simulink model "Motor_C_mex"  (R2024a)
settings: Solver=FixedStepAuto  StartTime=0.0  StopTime=20  FixedStep=MotorSampleTime  RelTol=1e-3
model workspace (MAT data in the model file):
  MotorSampleTime = 0.001
undefined symbols (not defined in the file): DiscIntNeverNeededParam
libraries: sldrtlib x1
settings Model: SimulationMode=accelerator  Creator=17739  LastModifiedBy=17739

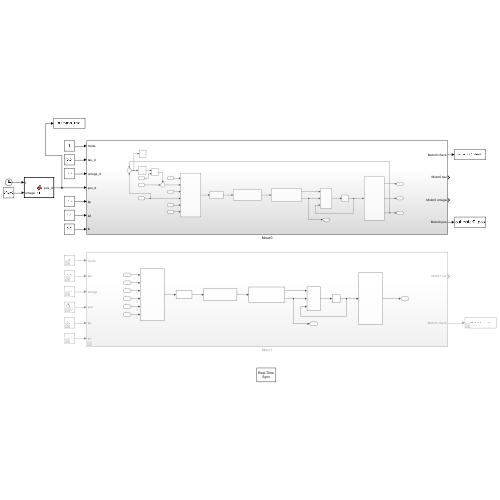
[thumbnail: Simulink's stored preview of the top-level diagram]
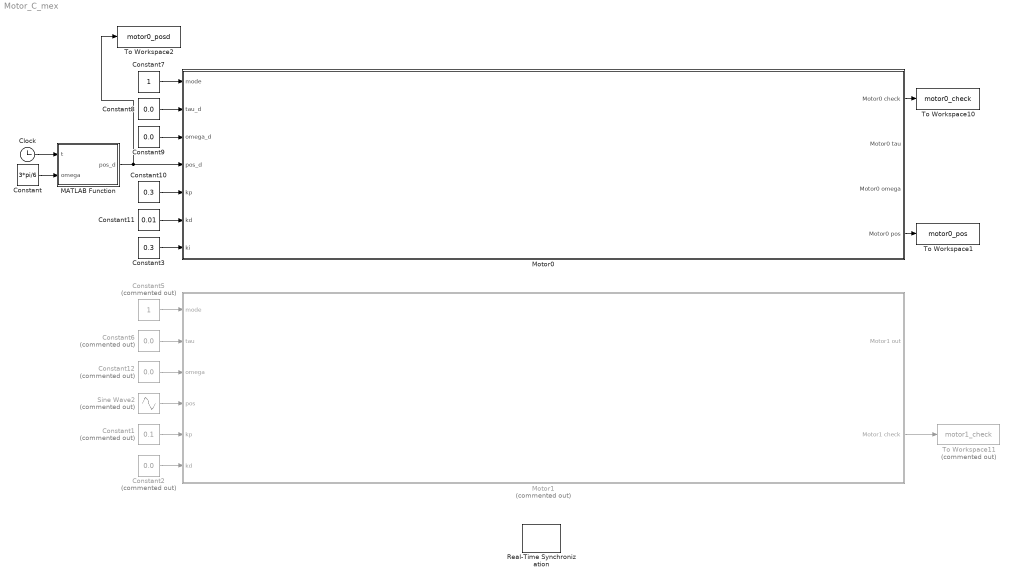
== system Motor_C_mex ==
  Clock : Clock
  Constant : Constant  Value=3*pi/6
  Constant1 : Constant  Commented=on  Value=0.1
  Constant10 : Constant  Value=0.3
  Constant11 : Constant  Value=0.01
  Constant12 : Constant  Commented=on  Value=0.0
  Constant2 : Constant  Commented=on  Value=0.0
  Constant3 : Constant  Value=0.3
  Constant5 : Constant  Commented=on
  Constant6 : Constant  Commented=on  Value=0.0
  Constant7 : Constant
  Constant8 : Constant  Value=0.0
  Constant9 : Constant  Value=0.0
  MATLAB Function : MATLAB Function  TreatAsAtomicUnit=on
  Motor0 : Subsystem
  Motor1 : Subsystem  Commented=on
  Real-Time Synchronization : sldrtlib/Real-Time Synchronization  SampleTime=MotorSampleTime  MaxMissedTicks=inf  ShowMissedTicks=off  YieldWhenWaiting=off
  Sine Wave2 : Sin  Commented=on  Amplitude=pi*6.33  Frequency=pi/5  SampleTime=MotorSampleTime
  To Workspace1 : ToWorkspace  VariableName=motor0_pos  SampleTime=-1
  To Workspace10 : ToWorkspace  VariableName=motor0_check  SampleTime=-1
  To Workspace11 : ToWorkspace  Commented=on  VariableName=motor1_check  SampleTime=-1
  To Workspace2 : ToWorkspace  VariableName=motor0_posd  SampleTime=-1
  wires:
  Constant7/1 -> Motor0/1(mode)
  Constant10/1 -> Motor0/5(kp)
  Motor1/2(Motor1 check) -> To Workspace11/1
  Constant8/1 -> Motor0/2(tau_d)
  Constant5/1 -> Motor1/1(mode)
  Constant2/1 -> Motor1/6(kd)
  Constant6/1 -> Motor1/2(tau)
  Constant11/1 -> Motor0/6(kd)
  Motor0/1(Motor0 check) -> To Workspace10/1
  Constant9/1 -> Motor0/3(omega_d)
  Constant1/1 -> Motor1/5(kp)
  Sine Wave2/1 -> Motor1/4(pos)
  Constant12/1 -> Motor1/3(omega)
  Constant3/1 -> Motor0/7(ki)
  Motor0/4(Motor0 pos) -> To Workspace1/1
  MATLAB Function/1(pos_d) -> To Workspace2/1, Motor0/4(pos_d)
  Clock/1 -> MATLAB Function/1(t)
  Constant/1 -> MATLAB Function/2(omega)

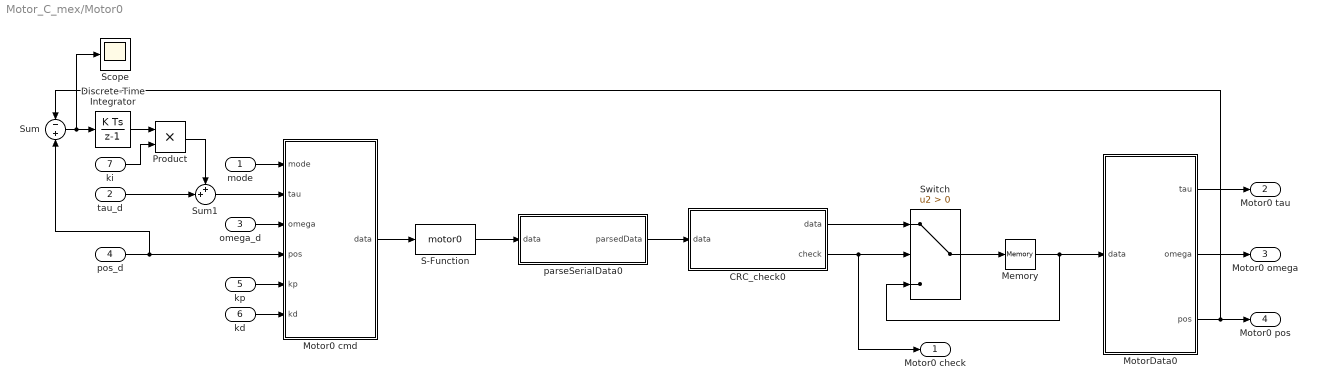
== system Motor_C_mex/Motor0 ==
  mode : Inport
  tau_d : Inport  Port=2
  omega_d : Inport  Port=3
  pos_d : Inport  Port=4
  kp : Inport  Port=5
  kd : Inport  Port=6
  ki : Inport  Port=7
  CRC_check0 : MATLAB Function  TreatAsAtomicUnit=on
  Discrete-Time Integrator : DiscreteIntegrator  SampleTime=-1  ICPrevOutput=DiscIntNeverNeededParam  ICPrevScaledInput=DiscIntNeverNeededParam
  Memory : Memory  InheritSampleTime=on
  Motor0 cmd : MATLAB Function  TreatAsAtomicUnit=on
  MotorData0 : MATLAB Function  TreatAsAtomicUnit=on
  Product : Product
  S-Function : S-Function  FunctionName=motor0  SFunctionDeploymentMode=off  EnableBusSupport=off
  Scope : Scope
  Sum : Sum  Inputs=-|+
  Sum1 : Sum  Inputs=++|
  Switch : Switch  Criteria=u2 > Threshold  SaturateOnIntegerOverflow=off  InputSameDT=off
  parseSerialData0 : MATLAB Function  TreatAsAtomicUnit=on
  Motor0 check : Outport
  Motor0 tau : Outport  Port=2
  Motor0 omega : Outport  Port=3
  Motor0 pos : Outport  Port=4
  wires:
  Motor0 cmd/1(data) -> S-Function/1
  parseSerialData0/1(parsedData) -> CRC_check0/1("data ")
  S-Function/1 -> parseSerialData0/1(data)
  Memory/1 -> MotorData0/1(data), Switch/3
  MotorData0/1(tau) -> Motor0 tau/1
  mode/1 -> Motor0 cmd/1(mode)
  Switch/1 -> Memory/1
  kd/1 -> Motor0 cmd/6(kd)
  CRC_check0/1(data) -> Switch/1
  CRC_check0/2(check) -> Motor0 check/1, Switch/2
  kp/1 -> Motor0 cmd/5(kp)
  omega_d/1 -> Motor0 cmd/3(omega)
  MotorData0/2(omega) -> Motor0 omega/1
  MotorData0/3(pos) -> Sum/1, Motor0 pos/1
  pos_d/1 -> Motor0 cmd/4(pos), Sum/2
  tau_d/1 -> Sum1/2
  Sum/1 -> Scope/1, Discrete-Time Integrator/1
  Discrete-Time Integrator/1 -> Product/1
  ki/1 -> Product/2
  Product/1 -> Sum1/1
  Sum1/1 -> Motor0 cmd/2(tau)

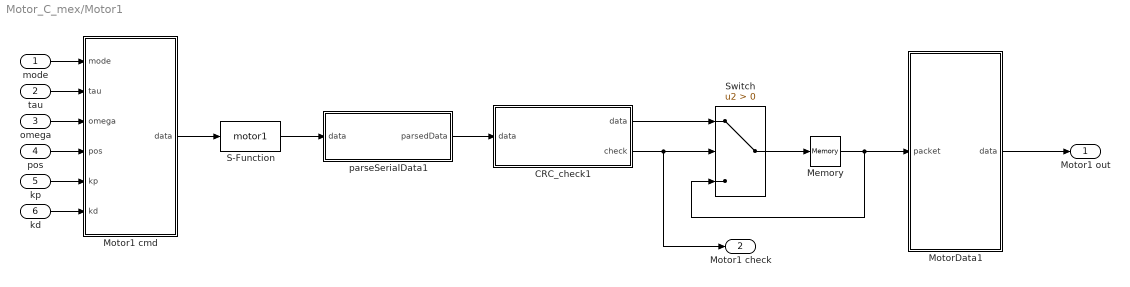
== system Motor_C_mex/Motor1 ==
  mode : Inport
  tau : Inport  Port=2
  omega : Inport  Port=3
  pos : Inport  Port=4
  kp : Inport  Port=5
  kd : Inport  Port=6
  CRC_check1 : MATLAB Function  TreatAsAtomicUnit=on
  Memory : Memory  InheritSampleTime=on
  Motor1 cmd : MATLAB Function  TreatAsAtomicUnit=on
  MotorData1 : MATLAB Function  TreatAsAtomicUnit=on
  S-Function : S-Function  FunctionName=motor1  SFunctionDeploymentMode=off  EnableBusSupport=off
  Switch : Switch  Criteria=u2 > Threshold  SaturateOnIntegerOverflow=off  InputSameDT=off
  parseSerialData1 : MATLAB Function  TreatAsAtomicUnit=on
  Motor1 out : Outport
  Motor1 check : Outport  Port=2
  wires:
  Motor1 cmd/1(data) -> S-Function/1
  parseSerialData1/1(parsedData) -> CRC_check1/1("data ")
  S-Function/1 -> parseSerialData1/1(data)
  Memory/1 -> MotorData1/1(packet), Switch/3
  Switch/1 -> Memory/1
  CRC_check1/1(data) -> Switch/1
  CRC_check1/2(check) -> Motor1 check/1, Switch/2
  omega/1 -> Motor1 cmd/3(omega)
  tau/1 -> Motor1 cmd/2(tau)
  pos/1 -> Motor1 cmd/4(pos)
  kp/1 -> Motor1 cmd/5(kp)
  kd/1 -> Motor1 cmd/6(kd)
  mode/1 -> Motor1 cmd/1(mode)
  MotorData1/1(data) -> Motor1 out/1

== matlab function Motor_C_mex/Motor1/CRC_check1 ==
  data: data output size=[1 16]; check output; data input
function [data, check] = CRC_Check(data)

crc_ccitt_table = [
    0x0000, 0x1189, 0x2312, 0x329b, 0x4624, 0x57ad, 0x6536, 0x74bf, ...
    0x8c48, 0x9dc1, 0xaf5a, 0xbed3, 0xca6c, 0xdbe5, 0xe97e, 0xf8f7, ...
    0x1081, 0x0108, 0x3393, 0x221a, 0x56a5, 0x472c, 0x75b7, 0x643e, ...
    0x9cc9, 0x8d40, 0xbfdb, 0xae52, 0xdaed, 0xcb64, 0xf9ff, 0xe876, ...
    0x2102, 0x308b, 0x0210, 0x1399, 0x6726, 0x76af, 0x4434, 0x55bd, ...
    0xad4a, 0xbcc3, 0x8e58, 0x9fd1, 0xeb6e, 0xfae7, 0xc87c, 0xd9f5, ...
    0x3183, 0x200a, 0x1291, 0x0318, 0x77a7, 0x662e, 0x54b5, 0x453c, ...
    0xbdcb, 0xac42, 0x9ed9, 0x8f50, 0xfbef, 0xea66, 0xd8fd, 0xc974, ...
    0x4204, 0x538d, 0x6116, 0x709f, 0x0420, 0x15a9, 0x2732, 0x36bb, ...
    0xce4c, 0xdfc5, 0xed5e, 0xfcd7, 0x8868, 0x99e1, 0xab7a, 0xbaf3, ...
    0x5285, 0x430c, 0x7197, 0x601e, 0x14a1, 0x0528, 0x37b3, 0x263a, ...
    0xdecd, 0xcf44, 0xfddf, 0xec56, 0x98e9, 0x8960, 0xbbfb, 0xaa72, ...
    0x6306, 0x728f, 0x4014, 0x519d, 0x2522, 0x34ab, 0x0630, 0x17b9, ...
    0xef4e, 0xfec7, 0xcc5c, 0xddd5, 0xa96a, 0xb8e3, 0x8a78, 0x9bf1, ...
    0x7387, 0x620e, 0x5095, 0x411c, 0x35a3, 0x242a, 0x16b1, 0x0738, ...
    0xffcf, 0xee46, 0xdcdd, 0xcd54, 0xb9eb, 0xa862, 0x9af9, 0x8b70, ...
    0x8408, 0x9581, 0xa71a, 0xb693, 0xc22c, 0xd3a5, 0xe13e, 0xf0b7, ...
    0x0840, 0x19c9, 0x2b52, 0x3adb, 0x4e64, 0x5fed, 0x6d76, 0x7cff, ...
    0x9489, 0x8500, 0xb79b, 0xa612, 0xd2ad, 0xc324, 0xf1bf, 0xe036, ...
    0x18c1, 0x0948, 0x3bd3, 0x2a5a, 0x5ee5, 0x4f6c, 0x7df7, 0x6c7e, ...
    0xa50a, 0xb483, 0x8618, 0x9791, 0xe32e, 0xf2a7, 0xc03c, 0xd1b5, ...
    0x2942, 0x38cb, 0x0a50, 0x1bd9, 0x6f66, 0x7eef, 0x4c74, 0x5dfd, ...
    0xb58b, 0xa402, 0x9699, 0x8710, 0xf3af, 0xe226, 0xd0bd, 0xc134, ...
    0x39c3, 0x284a, 0x1ad1, 0x0b58, 0x7fe7, 0x6e6e, 0x5cf5, 0x4d7c, ...
    0xc60c, 0xd785, 0xe51e, 0xf497, 0x8028, 0x91a1, 0xa33a, 0xb2b3, ...
    0x4a44, 0x5bcd, 0x6956, 0x78df, 0x0c60, 0x1de9, 0x2f72, 0x3efb, ...
    0xd68d, 0xc704, 0xf59f, 0xe416, 0x90a9, 0x8120, 0xb3bb, 0xa232, ...
    0x5ac5, 0x4b4c, 0x79d7, 0x685e, 0x1ce1, 0x0d68, 0x3ff3, 0x2e7a, ...
    0xe70e, 0xf687, 0xc41c, 0xd595, 0xa12a, 0xb0a3, 0x8238, 0x93b1, ...
    0x6b46, 0x7acf, 0x4854, 0x59dd, 0x2d62, 0x3ceb, 0x0e70, 0x1ff9, ...
    0xf78f, 0xe606, 0xd49d, 0xc514, 0xb1ab, 0xa022, 0x92b9, 0x8330, ...
    0x7bc7, 0x6a4e, 0x58d5, 0x495c, 0x3de3, 0x2c6a, 0x1ef1, 0x0f78 ...
    ];

crc = uint16(0);
for i = 1:14
    tableIndex = bitand(bitxor(crc, uint16(data(i))), uint16(0xff));
    crc = bitxor(bitshift(crc, -8), crc_ccitt_table(tableIndex + 1));
end
check = false;
if typecast(uint8(data(end-1:end)), 'uint16') == crc
    check = true;
end
end

== matlab function Motor_C_mex/Motor0/Motor0 cmd ==
  data: data output size=[1 17]; mode input; tau input; omega input; pos input; kp input; kd input
function data = MotorCmd(mode, tau, omega, pos, kp, kd)
data = uint8([hex2dec('FE'), hex2dec('EE'), ...
    mode*16 + 0, ...
    typecast(int16(fix(tau * 256)), 'uint8'), ...
    typecast(int16(fix(omega / (2 * pi) * 256)), 'uint8'), ...
    typecast(int32(fix(pos / (2 * pi) * 32768)), 'uint8'), ...
    typecast(int16(fix(kp * 1280)), 'uint8'), ...
    typecast(int16(fix(kd * 1280)), 'uint8'), ...
    0, 0]); % CRC16 计算稍后添加

% 计算并添加 CRC16 校验
crc = calculateCRC(data(1:15)); % 自定义 CRC 计算函数
data(16:17) = typecast(uint16(crc), 'uint8');
end
% 自定义 CRC 计算函数
function crc = calculateCRC(data)
crc_ccitt_table = [
    0x0000, 0x1189, 0x2312, 0x329b, 0x4624, 0x57ad, 0x6536, 0x74bf, ...
    0x8c48, 0x9dc1, 0xaf5a, 0xbed3, 0xca6c, 0xdbe5, 0xe97e, 0xf8f7, ...
    0x1081, 0x0108, 0x3393, 0x221a, 0x56a5, 0x472c, 0x75b7, 0x643e, ...
    0x9cc9, 0x8d40, 0xbfdb, 0xae52, 0xdaed, 0xcb64, 0xf9ff, 0xe876, ...
    0x2102, 0x308b, 0x0210, 0x1399, 0x6726, 0x76af, 0x4434, 0x55bd, ...
    0xad4a, 0xbcc3, 0x8e58, 0x9fd1, 0xeb6e, 0xfae7, 0xc87c, 0xd9f5, ...
    0x3183, 0x200a, 0x1291, 0x0318, 0x77a7, 0x662e, 0x54b5, 0x453c, ...
    0xbdcb, 0xac42, 0x9ed9, 0x8f50, 0xfbef, 0xea66, 0xd8fd, 0xc974, ...
    0x4204, 0x538d, 0x6116, 0x709f, 0x0420, 0x15a9, 0x2732, 0x36bb, ...
    0xce4c, 0xdfc5, 0xed5e, 0xfcd7, 0x8868, 0x99e1, 0xab7a, 0xbaf3, ...
    0x5285, 0x430c, 0x7197, 0x601e, 0x14a1, 0x0528, 0x37b3, 0x263a, ...
    0xdecd, 0xcf44, 0xfddf, 0xec56, 0x98e9, 0x8960, 0xbbfb, 0xaa72, ...
    0x6306, 0x728f, 0x4014, 0x519d, 0x2522, 0x34ab, 0x0630, 0x17b9, ...
    0xef4e, 0xfec7, 0xcc5c, 0xddd5, 0xa96a, 0xb8e3, 0x8a78, 0x9bf1, ...
    0x7387, 0x620e, 0x5095, 0x411c, 0x35a3, 0x242a, 0x16b1, 0x0738, ...
    0xffcf, 0xee46, 0xdcdd, 0xcd54, 0xb9eb, 0xa862, 0x9af9, 0x8b70, ...
    0x8408, 0x9581, 0xa71a, 0xb693, 0xc22c, 0xd3a5, 0xe13e, 0xf0b7, ...
    0x0840, 0x19c9, 0x2b52, 0x3adb, 0x4e64, 0x5fed, 0x6d76, 0x7cff, ...
    0x9489, 0x8500, 0xb79b, 0xa612, 0xd2ad, 0xc324, 0xf1bf, 0xe036, ...
    0x18c1, 0x0948, 0x3bd3, 0x2a5a, 0x5ee5, 0x4f6c, 0x7df7, 0x6c7e, ...
    0xa50a, 0xb483, 0x8618, 0x9791, 0xe32e, 0xf2a7, 0xc03c, 0xd1b5, ...
    0x2942, 0x38cb, 0x0a50, 0x1bd9, 0x6f66, 0x7eef, 0x4c74, 0x5dfd, ...
    0xb58b, 0xa402, 0x9699, 0x8710, 0xf3af, 0xe226, 0xd0bd, 0xc134, ...
    0x39c3, 0x284a, 0x1ad1, 0x0b58, 0x7fe7, 0x6e6e, 0x5cf5, 0x4d7c, ...
    0xc60c, 0xd785, 0xe51e, 0xf497, 0x8028, 0x91a1, 0xa33a, 0xb2b3, ...
    0x4a44, 0x5bcd, 0x6956, 0x78df, 0x0c60, 0x1de9, 0x2f72, 0x3efb, ...
    0xd68d, 0xc704, 0xf59f, 0xe416, 0x90a9, 0x8120, 0xb3bb, 0xa232, ...
    0x5ac5, 0x4b4c, 0x79d7, 0x685e, 0x1ce1, 0x0d68, 0x3ff3, 0x2e7a, ...
    0xe70e, 0xf687, 0xc41c, 0xd595, 0xa12a, 0xb0a3, 0x8238, 0x93b1, ...
    0x6b46, 0x7acf, 0x4854, 0x59dd, 0x2d62, 0x3ceb, 0x0e70, 0x1ff9, ...
    0xf78f, 0xe606, 0xd49d, 0xc514, 0xb1ab, 0xa022, 0x92b9, 0x8330, ...
    0x7bc7, 0x6a4e, 0x58d5, 0x495c, 0x3de3, 0x2c6a, 0x1ef1, 0x0f78 ...
    ];

crc = uint16(0);
for i = 1:length(data)
    tableIndex = bitand(bitxor(crc, uint16(data(i))), uint16(0xff));
    crc = bitxor(bitshift(crc, -8), crc_ccitt_table(tableIndex + 1));
end
end

== matlab function Motor_C_mex/Motor0/CRC_check0 ==
  data: data output size=[1 16]; check output; data input
function [data, check] = CRC_Check(data)

crc_ccitt_table = [
    0x0000, 0x1189, 0x2312, 0x329b, 0x4624, 0x57ad, 0x6536, 0x74bf, ...
    0x8c48, 0x9dc1, 0xaf5a, 0xbed3, 0xca6c, 0xdbe5, 0xe97e, 0xf8f7, ...
    0x1081, 0x0108, 0x3393, 0x221a, 0x56a5, 0x472c, 0x75b7, 0x643e, ...
    0x9cc9, 0x8d40, 0xbfdb, 0xae52, 0xdaed, 0xcb64, 0xf9ff, 0xe876, ...
    0x2102, 0x308b, 0x0210, 0x1399, 0x6726, 0x76af, 0x4434, 0x55bd, ...
    0xad4a, 0xbcc3, 0x8e58, 0x9fd1, 0xeb6e, 0xfae7, 0xc87c, 0xd9f5, ...
    0x3183, 0x200a, 0x1291, 0x0318, 0x77a7, 0x662e, 0x54b5, 0x453c, ...
    0xbdcb, 0xac42, 0x9ed9, 0x8f50, 0xfbef, 0xea66, 0xd8fd, 0xc974, ...
    0x4204, 0x538d, 0x6116, 0x709f, 0x0420, 0x15a9, 0x2732, 0x36bb, ...
    0xce4c, 0xdfc5, 0xed5e, 0xfcd7, 0x8868, 0x99e1, 0xab7a, 0xbaf3, ...
    0x5285, 0x430c, 0x7197, 0x601e, 0x14a1, 0x0528, 0x37b3, 0x263a, ...
    0xdecd, 0xcf44, 0xfddf, 0xec56, 0x98e9, 0x8960, 0xbbfb, 0xaa72, ...
    0x6306, 0x728f, 0x4014, 0x519d, 0x2522, 0x34ab, 0x0630, 0x17b9, ...
    0xef4e, 0xfec7, 0xcc5c, 0xddd5, 0xa96a, 0xb8e3, 0x8a78, 0x9bf1, ...
    0x7387, 0x620e, 0x5095, 0x411c, 0x35a3, 0x242a, 0x16b1, 0x0738, ...
    0xffcf, 0xee46, 0xdcdd, 0xcd54, 0xb9eb, 0xa862, 0x9af9, 0x8b70, ...
    0x8408, 0x9581, 0xa71a, 0xb693, 0xc22c, 0xd3a5, 0xe13e, 0xf0b7, ...
    0x0840, 0x19c9, 0x2b52, 0x3adb, 0x4e64, 0x5fed, 0x6d76, 0x7cff, ...
    0x9489, 0x8500, 0xb79b, 0xa612, 0xd2ad, 0xc324, 0xf1bf, 0xe036, ...
    0x18c1, 0x0948, 0x3bd3, 0x2a5a, 0x5ee5, 0x4f6c, 0x7df7, 0x6c7e, ...
    0xa50a, 0xb483, 0x8618, 0x9791, 0xe32e, 0xf2a7, 0xc03c, 0xd1b5, ...
    0x2942, 0x38cb, 0x0a50, 0x1bd9, 0x6f66, 0x7eef, 0x4c74, 0x5dfd, ...
    0xb58b, 0xa402, 0x9699, 0x8710, 0xf3af, 0xe226, 0xd0bd, 0xc134, ...
    0x39c3, 0x284a, 0x1ad1, 0x0b58, 0x7fe7, 0x6e6e, 0x5cf5, 0x4d7c, ...
    0xc60c, 0xd785, 0xe51e, 0xf497, 0x8028, 0x91a1, 0xa33a, 0xb2b3, ...
    0x4a44, 0x5bcd, 0x6956, 0x78df, 0x0c60, 0x1de9, 0x2f72, 0x3efb, ...
    0xd68d, 0xc704, 0xf59f, 0xe416, 0x90a9, 0x8120, 0xb3bb, 0xa232, ...
    0x5ac5, 0x4b4c, 0x79d7, 0x685e, 0x1ce1, 0x0d68, 0x3ff3, 0x2e7a, ...
    0xe70e, 0xf687, 0xc41c, 0xd595, 0xa12a, 0xb0a3, 0x8238, 0x93b1, ...
    0x6b46, 0x7acf, 0x4854, 0x59dd, 0x2d62, 0x3ceb, 0x0e70, 0x1ff9, ...
    0xf78f, 0xe606, 0xd49d, 0xc514, 0xb1ab, 0xa022, 0x92b9, 0x8330, ...
    0x7bc7, 0x6a4e, 0x58d5, 0x495c, 0x3de3, 0x2c6a, 0x1ef1, 0x0f78 ...
    ];

crc = uint16(0);
for i = 1:14
    tableIndex = bitand(bitxor(crc, uint16(data(i))), uint16(0xff));
    crc = bitxor(bitshift(crc, -8), crc_ccitt_table(tableIndex + 1));
end
check = false;
if typecast(uint8(data(end-1:end)), 'uint16') == crc
    check = true;
end
end

== matlab function Motor_C_mex/MATLAB Function ==
  data: t input; pos_d output; omega input
function pos_d = fcn(t, omega)
pos_d = (t-1)*omega*(t>=1 & t<7) + 6*omega*(t>=7 & t<11) + (17-t)*omega*(t>=11 & t<17);
end

== matlab function Motor_C_mex/Motor1/MotorData1 ==
  data: packet input; data output
function data = MotorData(packet)
data = zeros(1, 3);
data(1) = double(typecast(uint8(packet(4:5)), 'int16')) / 256; % tau
data(2) = double(typecast(uint8(packet(6:7)), 'int16')) / 256 * 2 * pi; % omega
data(3) = double(typecast(uint8(packet(8:11)), 'int32')) / 32768 * 2 * pi; % position
end

== matlab function Motor_C_mex/Motor1/parseSerialData1 ==
  data: data input; parsedData output
function parsedData = parseSerialData(data)
    persistent buffer0;
    if isempty(buffer0)
        buffer0 = uint8([]);
    end

    % Append new data to buffer, ensuring data is a row vector
    buffer0 = [buffer0, data(:)']; 

    % Define header and data size
    header = uint8([253, 238]); % 定义包头
    dataSize = 16; % 你的数据包大小

    % Initialize parsedData as an empty uint8 array of size 16
    parsedData = uint8([253, 238, zeros(1, dataSize-2)]);

    % Check if the buffer contains a valid packet
    while length(buffer0) >= dataSize
        % Find the header in the buffer
        headerPos = findHeader(buffer0, header);

        % If header is found and there is enough data for a full packet
        if ~isempty(headerPos) && (headerPos(1) + dataSize - 1 <= length(buffer0))
            % Extract the valid packet
            for num = 1:dataSize
                parsedData(num) = buffer0(headerPos(1) + num - 1);
            end
            % Remove the extracted packet from the buffer
            if length(headerPos) > 1
                buffer0 = buffer0(headerPos(2):end);
            else
                buffer0 = buffer0((headerPos(1) + dataSize):end);
            end
            return; % Exit the function after finding the first valid packet
        else
            % If no valid packet is found, clear the buffer up to the header position
            if ~isempty(headerPos)
                buffer0 = buffer0(headerPos(1):end);
            else
                buffer0 = uint8([]);
            end
            break;
        end
    end
end

function pos = findHeader(buffer, header)
    pos = [];
    for i = 1:(length(buffer) - length(header) + 1)
        if all(buffer(i:i + length(header) - 1) == header)
            pos = i;
            return;
        end
    end
end

== matlab function Motor_C_mex/Motor0/MotorData0 ==
  data: data input; tau output size=1; omega output size=1; pos output size=1
function [tau, omega, pos] = MotorData(data)
tau = double(typecast(uint8(data(4:5)), 'int16')) / 256;
omega = double(typecast(uint8(data(6:7)), 'int16')) / 256 * 2 * pi;
pos = double(typecast(uint8(data(8:11)), 'int32')) / 32768 * 2 * pi;
end

== matlab function Motor_C_mex/Motor0/parseSerialData0 ==
  data: data input; parsedData output size=[1, 16]
function parsedData = parseSerialData(data)
    persistent buffer0;
    if isempty(buffer0)
        buffer0 = uint8([]);
    end

    % Append new data to buffer, ensuring data is a row vector
    buffer0 = [buffer0, data(:)']; 

    % Define header and data size
    header = uint8([253, 238]); % 定义包头
    dataSize = 16; % 你的数据包大小

    % Initialize parsedData as an empty uint8 array of size 16
    parsedData = uint8([253, 238, zeros(1, dataSize-2)]);

    % Check if the buffer contains a valid packet
    while length(buffer0) >= dataSize
        % Find the header in the buffer
        headerPos = findHeader(buffer0, header);

        % If header is found and there is enough data for a full packet
        if ~isempty(headerPos) && (headerPos(1) + dataSize - 1 <= length(buffer0))
            % Extract the valid packet
            for num = 1:dataSize
                parsedData(num) = buffer0(headerPos(1) + num - 1);
            end
            % Remove the extracted packet from the buffer
            if length(headerPos) > 1
                buffer0 = buffer0(headerPos(2):end);
            else
                buffer0 = buffer0((headerPos(1) + dataSize):end);
            end
            return; % Exit the function after finding the first valid packet
        else
            % If no valid packet is found, clear the buffer up to the header position
            if ~isempty(headerPos)
                buffer0 = buffer0(headerPos(1):end);
            else
                buffer0 = uint8([]);
            end
            break;
        end
    end
end

function pos = findHeader(buffer, header)
    pos = [];
    for i = 1:(length(buffer) - length(header) + 1)
        if all(buffer(i:i + length(header) - 1) == header)
            pos = i;
            return;
        end
    end
end

== matlab function Motor_C_mex/Motor1/Motor1 cmd ==
  data: data output size=[1 17]; mode input; tau input; omega input; pos input; kp input; kd input
function data = MotorCmd(mode, tau, omega, pos, kp, kd)
data = uint8([hex2dec('FE'), hex2dec('EE'), ...
    mode*16 + 1, ...
    typecast(int16(fix(tau * 256)), 'uint8'), ...
    typecast(int16(fix(omega / (2 * pi) * 256)), 'uint8'), ...
    typecast(int32(fix(pos / (2 * pi) * 32768)), 'uint8'), ...
    typecast(int16(fix(kp * 1280)), 'uint8'), ...
    typecast(int16(fix(kd * 1280)), 'uint8'), ...
    0, 0]); % CRC16 计算稍后添加

% 计算并添加 CRC16 校验
crc = calculateCRC(data(1:15)); % 自定义 CRC 计算函数
data(16:17) = typecast(uint16(crc), 'uint8');
end
% 自定义 CRC 计算函数
function crc = calculateCRC(data)
crc_ccitt_table = [
    0x0000, 0x1189, 0x2312, 0x329b, 0x4624, 0x57ad, 0x6536, 0x74bf, ...
    0x8c48, 0x9dc1, 0xaf5a, 0xbed3, 0xca6c, 0xdbe5, 0xe97e, 0xf8f7, ...
    0x1081, 0x0108, 0x3393, 0x221a, 0x56a5, 0x472c, 0x75b7, 0x643e, ...
    0x9cc9, 0x8d40, 0xbfdb, 0xae52, 0xdaed, 0xcb64, 0xf9ff, 0xe876, ...
    0x2102, 0x308b, 0x0210, 0x1399, 0x6726, 0x76af, 0x4434, 0x55bd, ...
    0xad4a, 0xbcc3, 0x8e58, 0x9fd1, 0xeb6e, 0xfae7, 0xc87c, 0xd9f5, ...
    0x3183, 0x200a, 0x1291, 0x0318, 0x77a7, 0x662e, 0x54b5, 0x453c, ...
    0xbdcb, 0xac42, 0x9ed9, 0x8f50, 0xfbef, 0xea66, 0xd8fd, 0xc974, ...
    0x4204, 0x538d, 0x6116, 0x709f, 0x0420, 0x15a9, 0x2732, 0x36bb, ...
    0xce4c, 0xdfc5, 0xed5e, 0xfcd7, 0x8868, 0x99e1, 0xab7a, 0xbaf3, ...
    0x5285, 0x430c, 0x7197, 0x601e, 0x14a1, 0x0528, 0x37b3, 0x263a, ...
    0xdecd, 0xcf44, 0xfddf, 0xec56, 0x98e9, 0x8960, 0xbbfb, 0xaa72, ...
    0x6306, 0x728f, 0x4014, 0x519d, 0x2522, 0x34ab, 0x0630, 0x17b9, ...
    0xef4e, 0xfec7, 0xcc5c, 0xddd5, 0xa96a, 0xb8e3, 0x8a78, 0x9bf1, ...
    0x7387, 0x620e, 0x5095, 0x411c, 0x35a3, 0x242a, 0x16b1, 0x0738, ...
    0xffcf, 0xee46, 0xdcdd, 0xcd54, 0xb9eb, 0xa862, 0x9af9, 0x8b70, ...
    0x8408, 0x9581, 0xa71a, 0xb693, 0xc22c, 0xd3a5, 0xe13e, 0xf0b7, ...
    0x0840, 0x19c9, 0x2b52, 0x3adb, 0x4e64, 0x5fed, 0x6d76, 0x7cff, ...
    0x9489, 0x8500, 0xb79b, 0xa612, 0xd2ad, 0xc324, 0xf1bf, 0xe036, ...
    0x18c1, 0x0948, 0x3bd3, 0x2a5a, 0x5ee5, 0x4f6c, 0x7df7, 0x6c7e, ...
    0xa50a, 0xb483, 0x8618, 0x9791, 0xe32e, 0xf2a7, 0xc03c, 0xd1b5, ...
    0x2942, 0x38cb, 0x0a50, 0x1bd9, 0x6f66, 0x7eef, 0x4c74, 0x5dfd, ...
    0xb58b, 0xa402, 0x9699, 0x8710, 0xf3af, 0xe226, 0xd0bd, 0xc134, ...
    0x39c3, 0x284a, 0x1ad1, 0x0b58, 0x7fe7, 0x6e6e, 0x5cf5, 0x4d7c, ...
    0xc60c, 0xd785, 0xe51e, 0xf497, 0x8028, 0x91a1, 0xa33a, 0xb2b3, ...
    0x4a44, 0x5bcd, 0x6956, 0x78df, 0x0c60, 0x1de9, 0x2f72, 0x3efb, ...
    0xd68d, 0xc704, 0xf59f, 0xe416, 0x90a9, 0x8120, 0xb3bb, 0xa232, ...
    0x5ac5, 0x4b4c, 0x79d7, 0x685e, 0x1ce1, 0x0d68, 0x3ff3, 0x2e7a, ...
    0xe70e, 0xf687, 0xc41c, 0xd595, 0xa12a, 0xb0a3, 0x8238, 0x93b1, ...
    0x6b46, 0x7acf, 0x4854, 0x59dd, 0x2d62, 0x3ceb, 0x0e70, 0x1ff9, ...
    0xf78f, 0xe606, 0xd49d, 0xc514, 0xb1ab, 0xa022, 0x92b9, 0x8330, ...
    0x7bc7, 0x6a4e, 0x58d5, 0x495c, 0x3de3, 0x2c6a, 0x1ef1, 0x0f78 ...
    ];

crc = uint16(0);
for i = 1:length(data)
    tableIndex = bitand(bitxor(crc, uint16(data(i))), uint16(0xff));
    crc = bitxor(bitshift(crc, -8), crc_ccitt_table(tableIndex + 1));
end
end
